simulink model "DFIGStatorVoltageDrop"  (R2013a)
settings: Solver=ode8  StartTime=0.0  StopTime=3  FixedStep=0.0001  RelTol=1e-3
undefined symbols (not defined in the file): B, H, Xm, Xr, Z
libraries: powerlib x8
settings Model: Creator=Sony  LastModifiedBy=Sony

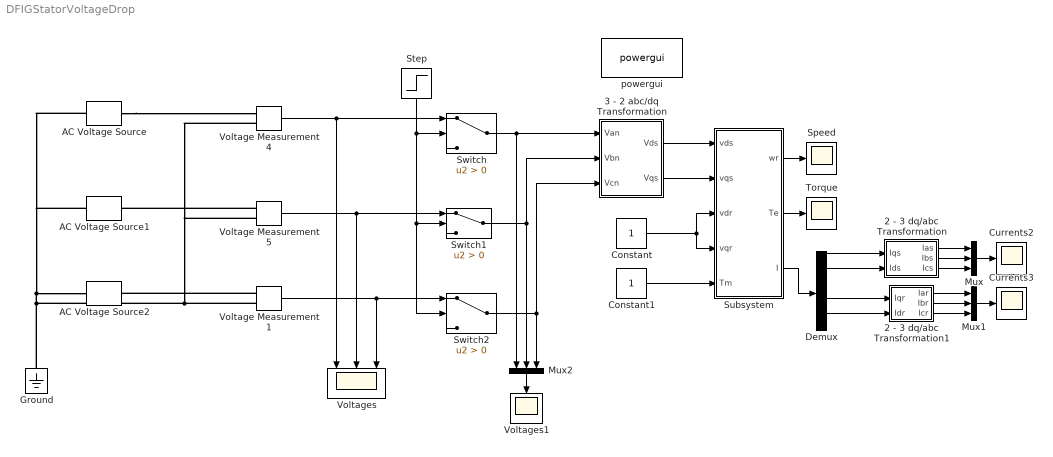
== system DFIGStatorVoltageDrop ==
  2 - 3 dq/abc Transformation : Subsystem
  2 - 3 dq/abc Transformation1 : Subsystem
  3 - 2 abc/dq Transformation : Subsystem
  AC Voltage Source : powerlib/Electrical Sources/AC Voltage Source  Amplitude=310.268700753  Phase=90  Frequency=50  SampleTime=0  Measurements=None
  AC Voltage Source1 : powerlib/Electrical Sources/AC Voltage Source  Amplitude=310.268700753  Phase=-30  Frequency=50  SampleTime=0  Measurements=None
  AC Voltage Source2 : powerlib/Electrical Sources/AC Voltage Source  Amplitude=310.268700753  Phase=-150  Frequency=50  SampleTime=0  Measurements=None
  Constant : Constant
  Constant1 : Constant
  Currents2 : Scope
      settings: SaveName=ScopeData2
  Currents3 : Scope
      settings: SaveName=ScopeData3
  Demux : Demux  Outputs=6
  Ground : powerlib/Elements/Ground  LConnTagsString=a
  Mux : Mux  Inputs=3
  Mux1 : Mux  Inputs=3
  Mux2 : Mux  Inputs=3
  Speed : Scope
      settings: SaveName=ScopeData4
  Step : Step  Time=2  Before=1  After=0  SampleTime=0
  Subsystem : Subsystem
  Switch : Switch  Criteria=u2 > Threshold
  Switch1 : Switch  Criteria=u2 > Threshold
  Switch2 : Switch  Criteria=u2 > Threshold
  Torque : Scope
      settings: SaveName=ScopeData5
  Voltage Measurement1 : powerlib/Measurements/Voltage Measurement  PhasorSimulation=off  OutputType=Complex  PSBequivalent=0
  Voltage Measurement4 : powerlib/Measurements/Voltage Measurement  PhasorSimulation=off  OutputType=Complex  PSBequivalent=0
  Voltage Measurement5 : powerlib/Measurements/Voltage Measurement  PhasorSimulation=off  OutputType=Complex  PSBequivalent=0
  Voltages : Scope  NumInputPorts=3
      settings: YMin=-5~-5~-5  YMax=5~5~5
  Voltages1 : Scope
  powergui : powerlib/powergui  Priority=1  SimulationMode=Continuous  SolverType=Tustin  SampleTime=50e-6  frequency=50  SPID=off  DisableSnubberDevices=off  DisableRonSwitches=off  DisableVfSwitches=off  SwTol=0  Interpol=off  DisplayEquations=off  frequencyindice=50  Pbase=100e6  ErrMax=1e-4  Iterations=50  UnitsV=kV  UnitsW=MW  FunctionMessages=off  echomessages=off  HookPort=off  EnableUseOfTLC=off  x0status=blocks  RestoreLinks=warning  ResistiveCurrentMeasurement=off  Frange=[0:2:500]  Ylog=off  Xlog=on  ShowGrid=off  save=off  variable=ZData  ZoomFFT=off  StartTime=0.0  cycles=1  DisplayStyle=1  fundamental=60  FreqAxis=off  MaxFrequency=1000  frequencyindicesteady=1  RmsSteady=1  display=off  Ts=0  methode=off
  wires:
  Voltage Measurement1/1 -> Switch2/1, Voltages/3
  Voltage Measurement5/1 -> Voltages/2, Switch1/1
  Switch/1 -> Mux2/1, 3 - 2 abc/dq Transformation/1(Van)
  Switch2/1 -> Mux2/3, 3 - 2 abc/dq Transformation/3(Vcn)
  Switch1/1 -> 3 - 2 abc/dq Transformation/2(Vbn), Mux2/2
  Step/1 -> Switch/2, Switch2/2, Switch1/2
  Voltage Measurement4/1 -> Switch/1, Voltages/1
  3 - 2 abc/dq Transformation/1(Vds) -> Subsystem/1(vds)
  3 - 2 abc/dq Transformation/2(Vqs) -> Subsystem/2(vqs)
  Subsystem/3(I) -> Demux/1
  Demux/1 -> 2 - 3 dq/abc Transformation/1(Iqs)
  Demux/2 -> 2 - 3 dq/abc Transformation/2(Ids)
  Demux/4 -> 2 - 3 dq/abc Transformation1/1(Iqr)
  Demux/5 -> 2 - 3 dq/abc Transformation1/2(Idr)
  2 - 3 dq/abc Transformation/1(Ias) -> Mux/1
  2 - 3 dq/abc Transformation/2(Ibs) -> Mux/2
  2 - 3 dq/abc Transformation/3(Ics) -> Mux/3
  2 - 3 dq/abc Transformation1/1(Iar) -> Mux1/1
  2 - 3 dq/abc Transformation1/2(Ibr) -> Mux1/2
  2 - 3 dq/abc Transformation1/3(Icr) -> Mux1/3
  Mux/1 -> Currents2/1
  Mux1/1 -> Currents3/1
  Constant/1 -> Subsystem/4(vqr), Subsystem/3(vdr)
  Subsystem/1(wr) -> Speed/1
  Subsystem/2(Te) -> Torque/1
  Mux2/1 -> Voltages1/1
  Constant1/1 -> Subsystem/5(Tm)
  connections:
  Voltage Measurement1/LConn2 -- Voltage Measurement5/LConn2 -- Voltage Measurement4/LConn2 -- Ground/LConn1 -- AC Voltage Source1/LConn1 -- AC Voltage Source/LConn1 -- AC Voltage Source2/LConn1
  AC Voltage Source/RConn1 -- Voltage Measurement4/LConn1
  Voltage Measurement1/LConn1 -- AC Voltage Source2/RConn1
  Voltage Measurement5/LConn1 -- AC Voltage Source1/RConn1

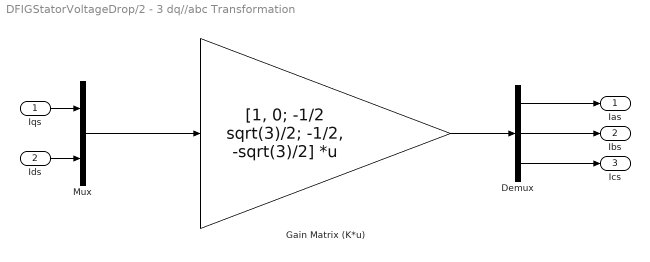
== system DFIGStatorVoltageDrop/2 - 3 dq//abc Transformation ==
  Iqs : Inport
  Ids : Inport  Port=2
  Demux : Demux  Outputs=3
  Gain Matrix (K*u) : Gain  Gain=[1, 0; -1/2 sqrt(3)/2; -1/2, -sqrt(3)/2]  Multiplication=Matrix(K*u)
  Mux : Mux  Inputs=2
  Ias : Outport
  Ibs : Outport  Port=2
  Ics : Outport  Port=3
  wires:
  Mux/1 -> Gain Matrix (K*u)/1
  Gain Matrix (K*u)/1 -> Demux/1
  Demux/2 -> Ibs/1
  Demux/1 -> Ias/1
  Demux/3 -> Ics/1
  Iqs/1 -> Mux/1
  Ids/1 -> Mux/2

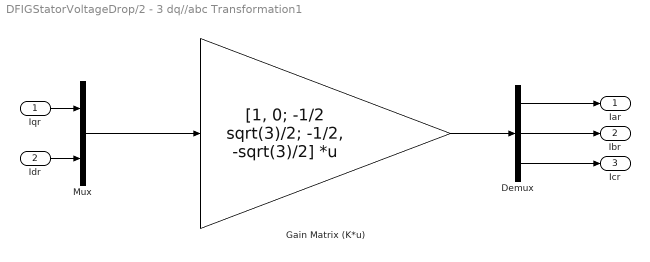
== system DFIGStatorVoltageDrop/2 - 3 dq//abc Transformation1 ==
  Iqr : Inport
  Idr : Inport  Port=2
  Demux : Demux  Outputs=3
  Gain Matrix (K*u) : Gain  Gain=[1, 0; -1/2 sqrt(3)/2; -1/2, -sqrt(3)/2]  Multiplication=Matrix(K*u)
  Mux : Mux  Inputs=2
  Iar : Outport
  Ibr : Outport  Port=2
  Icr : Outport  Port=3
  wires:
  Mux/1 -> Gain Matrix (K*u)/1
  Gain Matrix (K*u)/1 -> Demux/1
  Demux/2 -> Ibr/1
  Demux/1 -> Iar/1
  Demux/3 -> Icr/1
  Iqr/1 -> Mux/1
  Idr/1 -> Mux/2

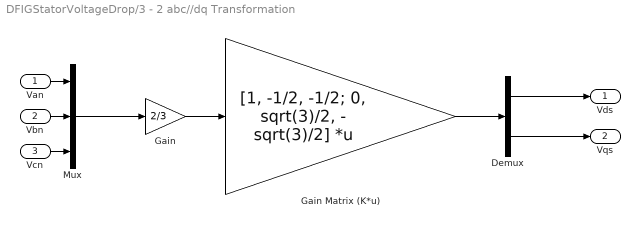
== system DFIGStatorVoltageDrop/3 - 2 abc//dq Transformation ==
  Van : Inport
  Vbn : Inport  Port=2
  Vcn : Inport  Port=3
  Demux : Demux  Outputs=2
  Gain : Gain  Gain=2/3
  Gain Matrix (K*u) : Gain  Gain=[1, -1/2, -1/2; 0, sqrt(3)/2, - sqrt(3)/2]  Multiplication=Matrix(K*u)
  Mux : Mux  Inputs=3
  Vds : Outport
  Vqs : Outport  Port=2
  wires:
  Vcn/1 -> Mux/3
  Vbn/1 -> Mux/2
  Van/1 -> Mux/1
  Gain/1 -> Gain Matrix (K*u)/1
  Gain Matrix (K*u)/1 -> Demux/1
  Mux/1 -> Gain/1
  Demux/1 -> Vds/1
  Demux/2 -> Vqs/1

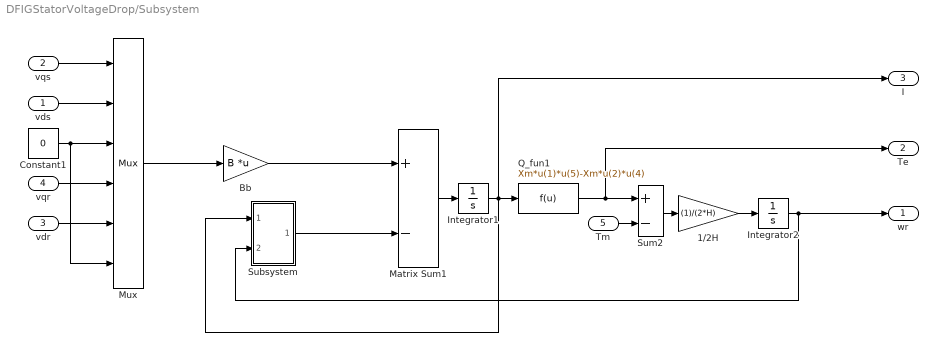
== system DFIGStatorVoltageDrop/Subsystem ==
  vds : Inport
  vqs : Inport  Port=2
  vdr : Inport  Port=3
  vqr : Inport  Port=4
  Tm : Inport  Port=5
  1/2H : Gain  Gain=(1)/(2*H)
  Bb : Gain  Gain=B  Multiplication=Matrix(K*u)
  Constant1 : Constant  Value=0
  Integrator1 : Integrator  InitialCondition=[0; 0; 0; 0; 0; 0]
  Integrator2 : Integrator
  Matrix Sum1 : Sum  Inputs=+-
  Mux : Mux  Inputs=6
  Q_fun1 : Fcn  Expr=Xm*u(1)*u(5)-Xm*u(2)*u(4)
  Subsystem : Subsystem
  Sum2 : Sum  Inputs=+-  SaturateOnIntegerOverflow=on  InputSameDT=on  OutDataTypeStr=Inherit: Same as first input
  wr : Outport
  Te : Outport  Port=2
  I : Outport  Port=3
  wires:
  Sum2/1 -> 1/2H/1
  vqs/1 -> Mux/1
  Matrix Sum1/1 -> Integrator1/1
  Constant1/1 -> Mux/6, Mux/3
  Tm/1 -> Sum2/2
  Q_fun1/1 -> Te/1, Sum2/1
  vds/1 -> Mux/2
  vdr/1 -> Mux/5
  Mux/1 -> Bb/1
  vqr/1 -> Mux/4
  1/2H/1 -> Integrator2/1
  Integrator1/1 -> Subsystem/1(In1), I/1, Q_fun1/1
  Bb/1 -> Matrix Sum1/1
  Integrator2/1 -> Subsystem/2(In2), wr/1
  Subsystem/1(Out1) -> Matrix Sum1/2

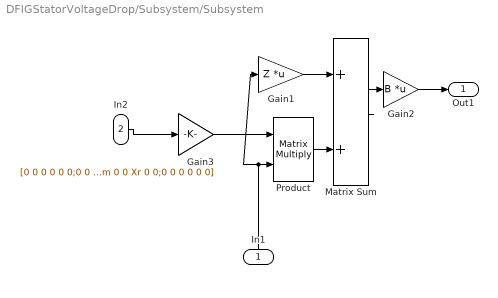
== system DFIGStatorVoltageDrop/Subsystem/Subsystem ==
  In1 : Inport
  In2 : Inport  Port=2
  Gain1 : Gain  Gain=Z  Multiplication=Matrix(K*u)
  Gain2 : Gain  Gain=B  Multiplication=Matrix(K*u)
  Gain3 : Gain  Gain=[0 0 0 0 0 0;0 0 0 0 0 0;0 0 0 0 0 0;0 -Xm 0 0 -Xr 0;Xm 0 0 Xr 0 0;0 0 0 0 0 0]
  Matrix Sum : Sum
  Product : Product  Multiplication=Matrix(*)
  Out1 : Outport
  wires:
  Gain2/1 -> Out1/1
  Product/1 -> Matrix Sum/2
  Matrix Sum/1 -> Gain2/1
  Gain3/1 -> Product/1
  Gain1/1 -> Matrix Sum/1
  In1/1 -> Gain1/1, Product/2
  In2/1 -> Gain3/1
